simulink model "Group1"  (R2024a)
settings: Solver=ode15s  StartTime=40000  StopTime=86400  MaxStep=1  RelTol=1e-5  AbsTol=1e-6
undefined symbols (not defined in the file or in its folder): J, Kd, Kf, Kg, Kt, L, R
libraries: slpidlib x2
settings Model: Creator=vishnu prasad  LastModifiedBy=vishnu prasad
settings SolverCC: MaxConsecutiveMinStep=50

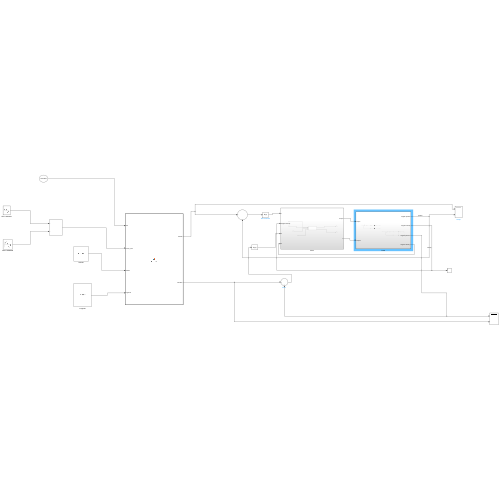
[thumbnail: Simulink's stored preview of the top-level diagram]
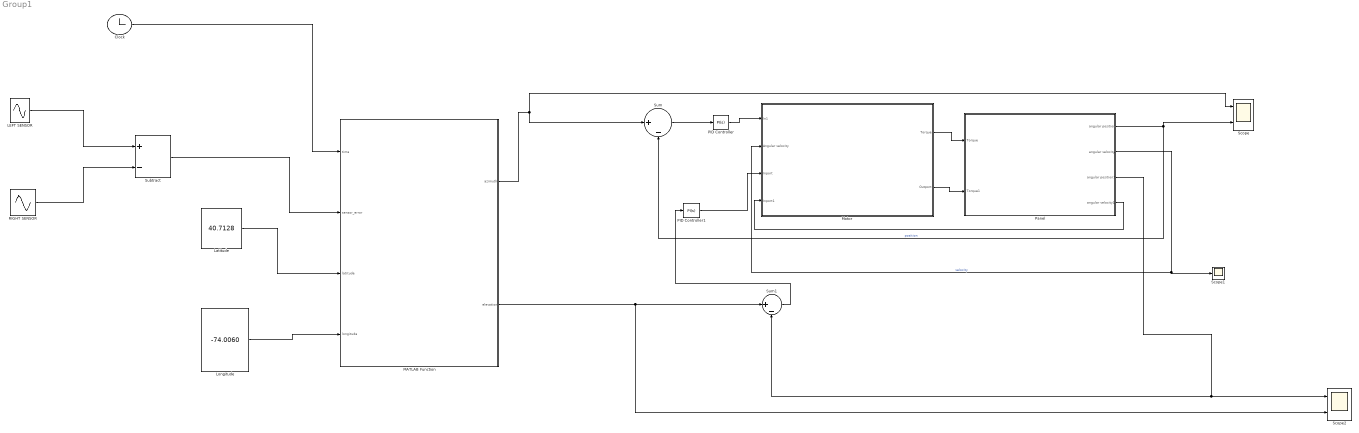
== system Group1 ==
  Clock : Clock
      settings: Decimation=86400*121
  LEFT SENSOR : Sin  Frequency=0.00004  SampleTime=0
  Latitude : Constant  Value=40.7128
  Longitude : Constant  Value=-74.0060
  MATLAB Function : MATLAB Function  TreatAsAtomicUnit=on
  Motor : Subsystem
  PID Controller : slpidlib/PID Controller  Controller=PI  Form=Parallel  TimeDomain=Continuous-time  UseExternalTs=off  SampleTime=-1  IntegratorMethod=Forward Euler  FilterMethod=Forward Euler  ControllerParametersSource=internal  P=240  I=180  UseKiTs=off  D=0  UseExternalDerivativeSource=off  N=100  UseFilter=on  TunerSelectOption=Transfer Function Based (PID Tuner App)  InitialConditionSource=internal  InitialConditionForIntegrator=0  InitialConditionForFilter=0  DifferentiatorICPrevScaledInput=0  ExternalReset=none  TrackingMode=off  Kt=1  LimitOutput=off  SatLimitsSource=internal  UpperSaturationLimit=inf  LowerSaturationLimit=-inf  LinearizeAsGain=on  AntiWindupMode=none  Kb=1  LimitIntegrator=off  UpperIntegratorSaturationLimit=inf  LowerIntegratorSaturationLimit=-inf  POutMin=[]  POutMax=[]  IOutMin=[]  IOutMax=[]  DOutMin=[]  DOutMax=[]  NOutMin=[]  NOutMax=[]  SumOutMin=[]  SumOutMax=[]  SaturationOutMin=[]  SaturationOutMax=[]  PParamMin=[]  PParamMax=[]  IParamMin=[]  IParamMax=[]  DParamMin=[]  DParamMax=[]  NParamMin=[]  NParamMax=[]  KbParamMin=[]  KbParamMax=[]  KtParamMin=[]  KtParamMax=[]  KbOutMin=[]  KbOutMax=[]  KtOutMin=[]  KtOutMax=[]  IntegratorOutMin=[]  IntegratorOutMax=[]  FilterOutMin=[]  FilterOutMax=[]  SumI1OutMin=[]  SumI1OutMax=[]  SumI2OutMin=[]  SumI2OutMax=[]  SumI3OutMin=[]  SumI3OutMax=[]  SumI4OutMin=[]  SumI4OutMax=[]  SumDOutMin=[]  SumDOutMax=[]  DifferentiatorOutMin=[]  DifferentiatorOutMax=[]  FilterDiffOutCoefMin=[]  FilterDiffOutCoefMax=[]  ReciprocalOutMin=[]  ReciprocalOutMax=[]  SumDenOutMin=[]  SumDenOutMax=[]  SumNumOutMin=[]  SumNumOutMax=[]  DivideOutMin=[]  DivideOutMax=[]  UdiffTsProdOutMin=[]  UdiffTsProdOutMax=[]  NTsProdOutMin=[]  NTsProdOutMax=[]  UintegralTsProdOutMin=[]  UintegralTsProdOutMax=[]  UngainTsProdOutMin=[]  UngainTsProdOutMax=[]  ClampingZeroOutDataTypeStr=Inherit: Inherit via back propagation  ClampingZeroOutMin=[]  ClampingZeroOutMax=[]  FilterDenConstantOutDataTypeStr=Inherit: Inherit via back propagation  FilterDenConstantOutMin=[]  FilterDenConstantOutMax=[]  PCopyOutDataTypeStr=Inherit: Inherit via back propagation  PCopyOutMin=[]  PCopyOutMax=[]  NCopyOutDataTypeStr=Inherit: Inherit via back propagation  NCopyOutMin=[]  NCopyOutMax=[]  IntegratorContinuousStateAttributes=''  IntegratorStateMustResolveToSignalObject=off  IntegratorRTWStateStorageClass=Auto  FilterContinuousStateAttributes=''  FilterStateMustResolveToSignalObject=off  FilterRTWStateStorageClass=Auto  ParallelPVariant=InternalParameters  IdealPVariant=Disabled  IVariant=InternalParameters  DVariant=Disabled  IntegratorVariant=Continuous  SatVariant=Disabled  AWVariant=Passthrough  PCopyVariant=Disabled  TRVariant=Disabled  FdbkBlocksVariant=Forward  IdealPFdbkVariant=Disabled  SatFdbkVariant=Disabled  DerivativeFilterVariant=Disabled  NVariant=Disabled  NCopyVariant=Disabled_SignalSpec  FilterICVariant=Disabled  IntegratorICVariant=InternalICs  ExternalResetVariant=Disabled  TRSumVariant=Passthrough  SumFdbkVariant=Disabled  SumVariant=Sum_PI  TsampFilterVariant=InternalTs  TsampNgainVariant=Passthrough  TsampIntegralVariant=Disabled_SignalSpec  ExternalSaturationOutDataTypeStr=Inherit: Same as second input  DerivativeSourceVariant=Disabled
  PID Controller1 : slpidlib/PID Controller  Controller=PI  Form=Parallel  TimeDomain=Continuous-time  UseExternalTs=off  SampleTime=-1  IntegratorMethod=Forward Euler  FilterMethod=Forward Euler  ControllerParametersSource=internal  P=240  I=180  UseKiTs=off  D=0  UseExternalDerivativeSource=off  N=100  UseFilter=on  TunerSelectOption=Transfer Function Based (PID Tuner App)  InitialConditionSource=internal  InitialConditionForIntegrator=0  InitialConditionForFilter=0  DifferentiatorICPrevScaledInput=0  ExternalReset=none  TrackingMode=off  Kt=1  LimitOutput=off  SatLimitsSource=internal  UpperSaturationLimit=inf  LowerSaturationLimit=-inf  LinearizeAsGain=on  AntiWindupMode=none  Kb=1  LimitIntegrator=off  UpperIntegratorSaturationLimit=inf  LowerIntegratorSaturationLimit=-inf  POutMin=[]  POutMax=[]  IOutMin=[]  IOutMax=[]  DOutMin=[]  DOutMax=[]  NOutMin=[]  NOutMax=[]  SumOutMin=[]  SumOutMax=[]  SaturationOutMin=[]  SaturationOutMax=[]  PParamMin=[]  PParamMax=[]  IParamMin=[]  IParamMax=[]  DParamMin=[]  DParamMax=[]  NParamMin=[]  NParamMax=[]  KbParamMin=[]  KbParamMax=[]  KtParamMin=[]  KtParamMax=[]  KbOutMin=[]  KbOutMax=[]  KtOutMin=[]  KtOutMax=[]  IntegratorOutMin=[]  IntegratorOutMax=[]  FilterOutMin=[]  FilterOutMax=[]  SumI1OutMin=[]  SumI1OutMax=[]  SumI2OutMin=[]  SumI2OutMax=[]  SumI3OutMin=[]  SumI3OutMax=[]  SumI4OutMin=[]  SumI4OutMax=[]  SumDOutMin=[]  SumDOutMax=[]  DifferentiatorOutMin=[]  DifferentiatorOutMax=[]  FilterDiffOutCoefMin=[]  FilterDiffOutCoefMax=[]  ReciprocalOutMin=[]  ReciprocalOutMax=[]  SumDenOutMin=[]  SumDenOutMax=[]  SumNumOutMin=[]  SumNumOutMax=[]  DivideOutMin=[]  DivideOutMax=[]  UdiffTsProdOutMin=[]  UdiffTsProdOutMax=[]  NTsProdOutMin=[]  NTsProdOutMax=[]  UintegralTsProdOutMin=[]  UintegralTsProdOutMax=[]  UngainTsProdOutMin=[]  UngainTsProdOutMax=[]  ClampingZeroOutDataTypeStr=Inherit: Inherit via back propagation  ClampingZeroOutMin=[]  ClampingZeroOutMax=[]  FilterDenConstantOutDataTypeStr=Inherit: Inherit via back propagation  FilterDenConstantOutMin=[]  FilterDenConstantOutMax=[]  PCopyOutDataTypeStr=Inherit: Inherit via back propagation  PCopyOutMin=[]  PCopyOutMax=[]  NCopyOutDataTypeStr=Inherit: Inherit via back propagation  NCopyOutMin=[]  NCopyOutMax=[]  IntegratorContinuousStateAttributes=''  IntegratorStateMustResolveToSignalObject=off  IntegratorRTWStateStorageClass=Auto  FilterContinuousStateAttributes=''  FilterStateMustResolveToSignalObject=off  FilterRTWStateStorageClass=Auto  ParallelPVariant=InternalParameters  IdealPVariant=Disabled  IVariant=InternalParameters  DVariant=Disabled  IntegratorVariant=Continuous  SatVariant=Disabled  AWVariant=Passthrough  PCopyVariant=Disabled  TRVariant=Disabled  FdbkBlocksVariant=Forward  IdealPFdbkVariant=Disabled  SatFdbkVariant=Disabled  DerivativeFilterVariant=Disabled  NVariant=Disabled  NCopyVariant=Disabled_SignalSpec  FilterICVariant=Disabled  IntegratorICVariant=InternalICs  ExternalResetVariant=Disabled  TRSumVariant=Passthrough  SumFdbkVariant=Disabled  SumVariant=Sum_PI  TsampFilterVariant=InternalTs  TsampNgainVariant=Passthrough  TsampIntegralVariant=Disabled_SignalSpec  ExternalSaturationOutDataTypeStr=Inherit: Same as second input  DerivativeSourceVariant=Disabled
  Panel : Subsystem
  RIGHT SENSOR : Sin  Frequency=0.00004  SampleTime=0
  Scope : Scope  NumInputPorts=2
  Scope1 : Scope
  Scope2 : Scope  NumInputPorts=2
  Subtract : Sum  Inputs=+-
  Sum : Sum  Inputs=|+-
  Sum1 : Sum  Inputs=|+-
  wires:
  Panel/3(angular position1) -> Sum1/2, Scope2/1
  Panel/2(angular velocity) -> Scope1/1, Motor/2(Angular velocity)  "velocity"
  Panel/1(angular position) -> Scope/2, Sum/2  "position"
  PID Controller/1 -> Motor/1(In1)
  Sum1/1 -> PID Controller1/1
  Motor/1(Torque) -> Panel/1(Torque)
  Clock/1 -> MATLAB Function/1(time)
  Sum/1 -> PID Controller/1
  Motor/2(Outport) -> Panel/2(Torque1)
  MATLAB Function/2(elevation) -> Scope2/2, Sum1/1
  PID Controller1/1 -> Motor/3(Inport)
  Panel/4(angular velocity1) -> Motor/4(Inport1)
  LEFT SENSOR/1 -> Subtract/1
  RIGHT SENSOR/1 -> Subtract/2
  MATLAB Function/1(azimuth) -> Sum/1, Scope/1
  Latitude/1 -> MATLAB Function/3(latitude)
  Longitude/1 -> MATLAB Function/4(longitude)
  Subtract/1 -> MATLAB Function/2(sensor_error)

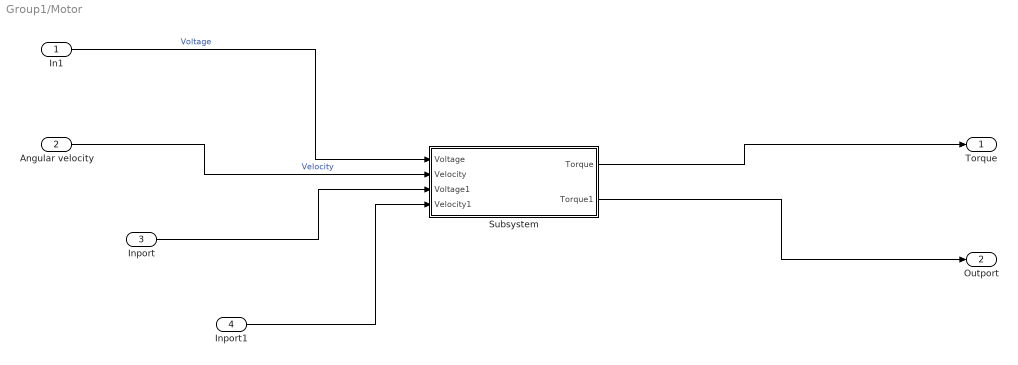
== system Group1/Motor ==
  In1 : Inport
  Angular velocity : Inport  Port=2
  Inport : Inport  Port=3
  Inport1 : Inport  Port=4
  Subsystem : Subsystem
  Torque : Outport
  Outport : Outport  Port=2
  wires:
  In1/1 -> Subsystem/1(Voltage)  "Voltage"
  Angular velocity/1 -> Subsystem/2(Velocity)  "Velocity"
  Subsystem/1(Torque) -> Torque/1
  Inport/1 -> Subsystem/3(Voltage1)
  Inport1/1 -> Subsystem/4(Velocity1)
  Subsystem/2(Torque1) -> Outport/1

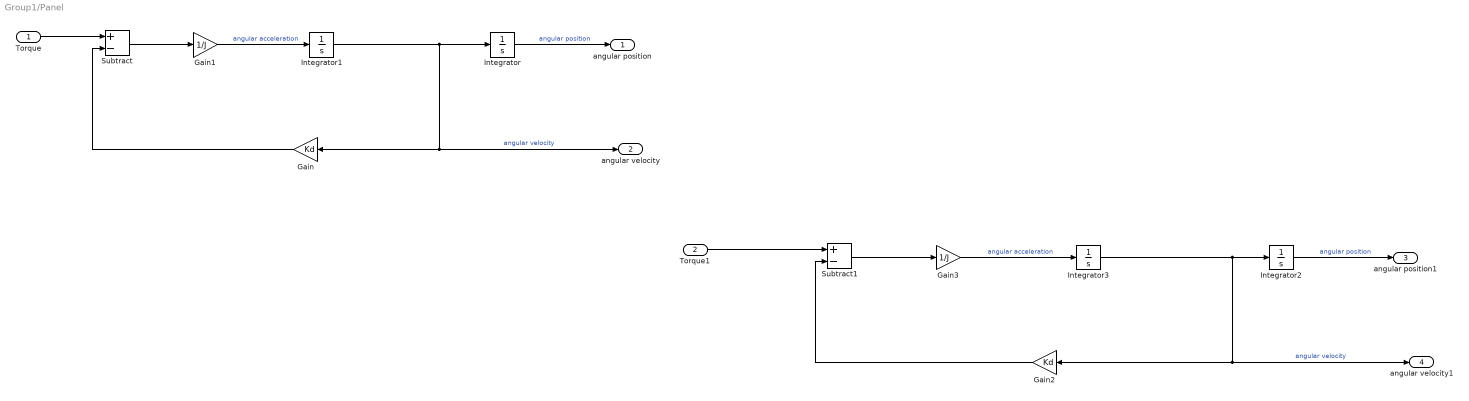
== system Group1/Panel ==
  Torque : Inport
  Torque1 : Inport  Port=2
  Gain : Gain  Gain=Kd
  Gain1 : Gain  Gain=1/J
  Gain2 : Gain  Gain=Kd
  Gain3 : Gain  Gain=1/J
  Integrator{,1..3} (4 alike) : Integrator
  Subtract : Sum  Inputs=+-
  Subtract1 : Sum  Inputs=+-
  angular position : Outport
  angular velocity : Outport  Port=2
  angular position1 : Outport  Port=3
  angular velocity1 : Outport  Port=4
  wires:
  Integrator/1 -> angular position/1  "angular position"
  Torque/1 -> Subtract/1
  Integrator1/1 -> Integrator/1, angular velocity/1, Gain/1  "angular velocity"
  Gain/1 -> Subtract/2
  Gain1/1 -> Integrator1/1  "angular acceleration"
  Subtract/1 -> Gain1/1
  Integrator2/1 -> angular position1/1  "angular position"
  Integrator3/1 -> angular velocity1/1, Gain2/1, Integrator2/1  "angular velocity"
  Gain3/1 -> Integrator3/1  "angular acceleration"
  Gain2/1 -> Subtract1/2
  Torque1/1 -> Subtract1/1
  Subtract1/1 -> Gain3/1

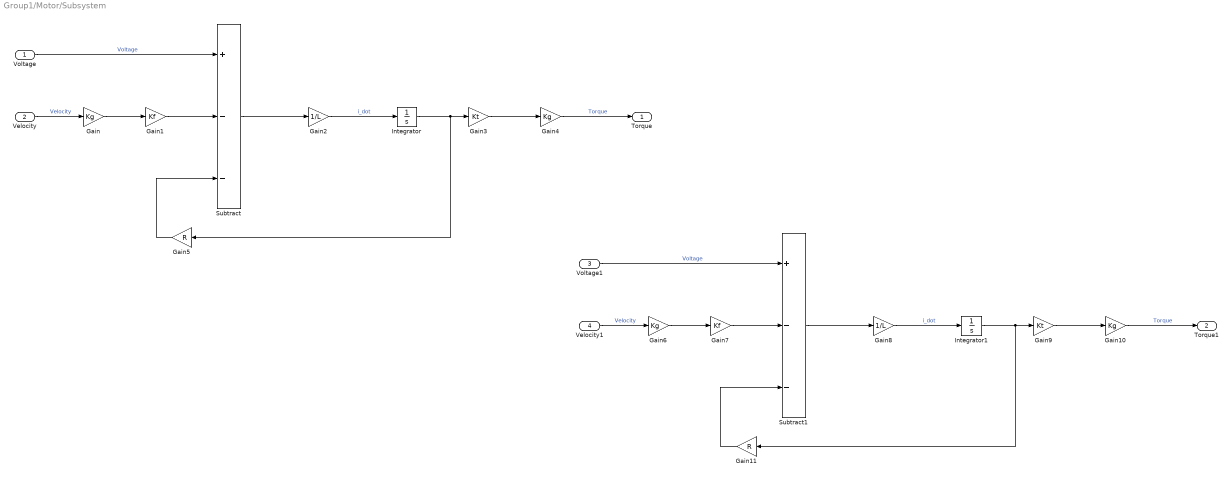
== system Group1/Motor/Subsystem ==
  Voltage : Inport
  Velocity : Inport  Port=2
  Voltage1 : Inport  Port=3
  Velocity1 : Inport  Port=4
  Gain{,4,6,10} (4 alike) : Gain  Gain=Kg
  Gain1 : Gain  Gain=Kf
  Gain11 : Gain  Gain=R
  Gain2 : Gain  Gain=1/L
  Gain3 : Gain  Gain=Kt
  Gain5 : Gain  Gain=R
  Gain7 : Gain  Gain=Kf
  Gain8 : Gain  Gain=1/L
  Gain9 : Gain  Gain=Kt
  Integrator : Integrator
  Integrator1 : Integrator
  Subtract : Sum  Inputs=+--
  Subtract1 : Sum  Inputs=+--
  Torque : Outport
  Torque1 : Outport  Port=2
  wires:
  Gain3/1 -> Gain4/1
  Gain1/1 -> Subtract/2
  Gain2/1 -> Integrator/1  "i_dot"
  Integrator/1 -> Gain5/1, Gain3/1
  Gain/1 -> Gain1/1
  Gain4/1 -> Torque/1  "Torque"
  Gain5/1 -> Subtract/3
  Velocity/1 -> Gain/1  "Velocity"
  Subtract/1 -> Gain2/1
  Voltage/1 -> Subtract/1  "Voltage"
  Voltage1/1 -> Subtract1/1  "Voltage"
  Subtract1/1 -> Gain8/1
  Velocity1/1 -> Gain6/1  "Velocity"
  Integrator1/1 -> Gain11/1, Gain9/1
  Gain11/1 -> Subtract1/3
  Gain10/1 -> Torque1/1  "Torque"
  Gain8/1 -> Integrator1/1  "i_dot"
  Gain9/1 -> Gain10/1
  Gain7/1 -> Subtract1/2
  Gain6/1 -> Gain7/1

== matlab function Group1/MATLAB Function ==
  data: time input; azimuth output; elevation output; sensor_error input; latitude input; longitude input
function [azimuth, elevation] = sun_path(time, sensor_error, latitude, longitude)
    % Constants
    dayLength = 86400; % Total seconds in a day (24*60*60)
    
    % Normalize time to a 24-hour period
    normalizedTime = mod(time, dayLength) / dayLength;
    
    % Solar declination angle (simplified)
    declination = 23.45 * sind(2 * pi * (284 + time / 86400 * 365.25) / 365);
    
    % Hour angle
    hourAngle = (normalizedTime - 0.5) * 360 + longitude;
    
    % Elevation angle (simplified)
    elevation = asind(sind(latitude) * sind(declination) + ...
                      cosd(latitude) * cosd(declination) * cosd(hourAngle));
    
    % Azimuth angle (simplified)
    if elevation > 0
        azimuth = acosd((sind(declination) - sind(elevation) * sind(latitude)) / ...
                        (cosd(elevation) * cosd(latitude)));
        if hourAngle > 0
            azimuth = 360 - azimuth;
        end
    else
        azimuth = 0; % Sun below horizon
    end
    
    % Adjust azimuth based on sensor error
    % Assuming sensor_error is in degrees and affects azimuth directly
    azimuth = azimuth + sensor_error;
    
    % Ensure azimuth is within the valid range [0, 360]
    if azimuth < 0
        azimuth = azimuth + 360;
    elseif azimuth >= 360
        azimuth = azimuth - 360;
    end
    
    % Convert angles to radians if needed
    azimuth = deg2rad(azimuth);
    elevation = deg2rad(elevation);
end
